simulink model "VTOL_aircraft_model"  (R2019b)
settings: Solver=FixedStepAuto  StartTime=0.0  StopTime=20  FixedStep=0.001  RelTol=1e-3
settings Model: Creator=陈冠军  LastModifiedBy=陈冠军

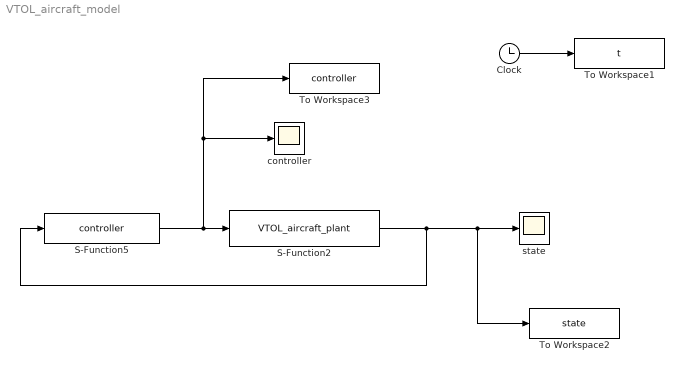
== system VTOL_aircraft_model ==
  Clock : Clock
      settings: Decimation=40
  S-Function2 : S-Function  FunctionName=VTOL_aircraft_plant  Parameters=iniState  SFunctionDeploymentMode=off  EnableBusSupport=off  mask{iniState=[5,0.1,-5,-0.1,pi,0.1]}
  S-Function5 : S-Function  FunctionName=controller  SFunctionDeploymentMode=off  EnableBusSupport=off
  To Workspace1 : ToWorkspace  VariableName=t  SampleTime=-1
  To Workspace2 : ToWorkspace  VariableName=state  SampleTime=-1
  To Workspace3 : ToWorkspace  VariableName=controller  SampleTime=-1
  controller : Scope
  state : Scope
  wires:
  Clock/1 -> To Workspace1/1
  S-Function2/1 -> S-Function5/1, To Workspace2/1, state/1
  S-Function5/1 -> To Workspace3/1, controller/1, S-Function2/1
